simulink model "VSC_GFo_Fixed_Frequency_LCL"  (R2017a)
settings: Solver=ode1  StartTime=0.0  StopTime=15  FixedStep=Time_Step  MaxStep=1e-5  RelTol=1e-3
PreLoadFcn:
  | VSC_GFo_Init;
InitFcn:
  | VSC_GFo_Init;
undefined symbols (not defined in the file): fb, GRD00_H, GRD00_R, GRD00_TD, GRD00_TN, GRD00_Ub, L_1, L_2, R_1, R_2, Time_Step, VSC01_Delta_P_Time_Step, VSC01_Delta_P_Value
libraries: powerlib x14, Source_Lib x1, GFo_Lib x1
settings Model: Creator=Frederic_Colas  LastModifiedBy=Frederic_Colas
settings DataIOCC: SaveFormat=StructureWithTime
settings OptimizationCC: LifeSpan=inf
settings DebuggingCC: UnconnectedInputMsg=none  UnconnectedOutputMsg=none  UnconnectedLineMsg=none  SFExecutionAtInitializationDiag=none
settings HardwareCC: ProdBitPerSizeT=32  ProdBitPerPtrDiffT=32  ProdWordSize=32  ProdHWDeviceType=Specified
settings SimscapeCC: SimscapeNormalizeSystem=off

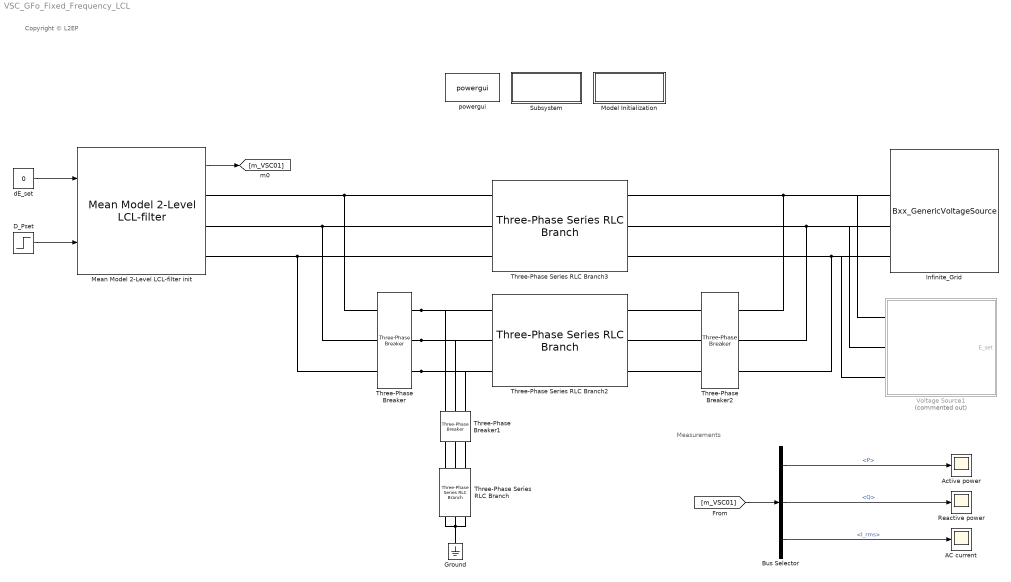
== system VSC_GFo_Fixed_Frequency_LCL ==
  note: Copyright © L2EP
  note: Measurements
  AC current : Scope
  Active power : Scope
  Bus Selector : BusSelector  OutputSignals=control.P,control.Q,control.VI.I_rms
  D_Pset : Step  Time=VSC01_Delta_P_Time_Step  After=VSC01_Delta_P_Value  SampleTime=0
  Ground : powerlib/Elements/Ground  LConnTagsString=a
  Infinite_Grid : Source_Lib/Bxx_GenericVoltageSource  SourceNature_str=INFINITE  fn=50  Sn=1e9  Un=400e3  LFpopup=Swing  P0=-778001534.1192  Q0=217439550.3985  V0_pu=1  U0=20000  Theta0_deg=0  H_s=5  DroopOnOff=on  R_percent=4  TN=1  TD=2
      settings: SourceProductName=VSC4SPS
  Mean Model 2-Level LCL-filter init : GFo_Lib/Mean Model 2-Level LCL-filter  fn=fn  Sn=VSC01_Sn  Pn=VSC01_Pn  Udcn=VSC01_Udc_n  Un1=VSC01_Un1  Un2=VSC01_Un2  Rt_pu=0.005  Lt_pu=0.15  Rm_pu=500  Lm_pu=500  Lf_pu=0.15  Rf_pu=0.005  Cf_pu=0.066  Tr_PLL=10e-3  Val_Freq_Support=on  Val_gamma=on  R_percent=4  Rv=0.009  W_TVR=60  I_thresh_pu=1  DX_DR=5  Kp_Rvi_pu=0.676  gainpopup=3  wc1=31.4159  mp1=0.0043  wc2=33.3  mp2=0.0033  wc3=2.5  mp3=0.04  T1=0.1210  T2=0.022  LFpopup=PQ  P0=0.79991  Q0=0.00012364  V0=0.99007  Theta0=15.6198  innercontrol=1  Kp_i=0.73/2  Ki_i=1.19/2  Kp_v=0.52  Ki_v=1.16  Kffv=1  Kffi=1  I_max=1.25
      settings: SourceProductName=VSC_Lib
  Model Initialization : Subsystem  mask(Model Functions){InitFcnX=VSC_GFo_Init;, prel=on, posl=off, inif=on, strf=off}
      mask prompts: InitFcnX "Initialisation"; prel "Preload Function"; posl "PostLoad Function"; inif "InitFcn"; strf "StartFcn"
      mask init:
      | currentBlock = gcb;
      | root = bdroot(currentBlock);
      | 
      | if ~strcmp(get_param(root,'BlockDiagramType'),'library')
      |     if prel==1
      |         set_param(root, 'PreLoadFcn', InitFcnX);
      |     else
      |         set_param(root, 'PreLoadFcn', '');
      |     end
      |     if inif==1
      |         set_param(root, 'InitFcn', InitFcnX);
      |     else
      |         set_param(root, 'InitFcn', '');
      |     end
      |     if strf==1
      |         set_param(root, 'StartFcn', InitFcnX);
      |     else
      |         set_param(root, 'StartFcn', '');
      |     end
      |     if posl==1
      |         set_param(root, 'PostLoadFcn', InitFcnX);
      |     else
      |         set_param(root, 'PostLoadFcn', '');
      |     end
      | end
      | 
      | pos = get_param(currentBlock, 'Position');
      | width = pos(3) - pos(1); height = pos(4) - pos(2);
      | txt = [ upper(root) '\n' '- InitFcn. . . . . '  get_param(root, 'InitFcn') ];
      settings: CopyFcn=set_param(gcb,'LinkStatus','none')
      mask Display:
      | %text(5, height*0.5, txt, 'horizontalAlignment', 'left', 'verticalAlignment', 'middle') ;
      | color('blue'),disp('Initialization Function\nParameters')
  Reactive power : Scope
  Subsystem : Subsystem
      settings: OpenFcn=LoadFlow_VSC
      mask Display: color('blue'),disp('Update Loadflow')
  Three-Phase Series RLC Branch : powerlib/Elements/Three-Phase Series RLC Branch  LConnTagsString=A|B|C  RConnTagsString=A|B|C  BranchType=R  Resistance=0.01  Inductance=1e-3  Capacitance=1e-6  Measurements=None
  Three-Phase Series RLC Branch2 : powerlib/Elements/Three-Phase Series RLC Branch  LConnTagsString=A|B|C  RConnTagsString=A|B|C  BranchType=RL  Resistance=R_2  Inductance=L_2  Capacitance=1e-6  Measurements=None
  Three-Phase Series RLC Branch3 : powerlib/Elements/Three-Phase Series RLC Branch  LConnTagsString=A|B|C  RConnTagsString=A|B|C  BranchType=RL  Resistance=R_1  Inductance=L_1  Capacitance=1e-6  Measurements=None
  Three-Phase Breaker : powerlib/Elements/Three-Phase Breaker  InitialState=closed  SwitchA=on  SwitchB=on  SwitchC=on  SwitchTimes=[1.5 4]  External=off  BreakerResistance=0.01  SnubberResistance=1e6  SnubberCapacitance=inf  Measurements=None
  Three-Phase Breaker1 : powerlib/Elements/Three-Phase Breaker  InitialState=open  SwitchA=on  SwitchB=on  SwitchC=on  SwitchTimes=[10 10.2]  External=off  BreakerResistance=0.01  SnubberResistance=1e6  SnubberCapacitance=inf  Measurements=None
  Three-Phase Breaker2 : powerlib/Elements/Three-Phase Breaker  InitialState=closed  SwitchA=on  SwitchB=on  SwitchC=on  SwitchTimes=[1.5 4]  External=off  BreakerResistance=0.01  SnubberResistance=1e6  SnubberCapacitance=inf  Measurements=None
  Voltage Source1 : Subsystem  Commented=on  mask(Fixed_source){fb=fb, Sc=1e9, Ub=GRD00_Ub, H_eq=GRD00_H, Droop=GRD00_R, TN=GRD00_TN, TD=GRD00_TD}
      mask prompts: fb "Nominal Frequency (Hz)"; Sc "Nominal Power (VA)"; Ub "Nominal Voltage (V)"; H_eq "Inertial Constant H (s)"; Droop "Droop Gain"; TN "Lead Time Constant"; TD "Lag Time Constant"
      mask init:
      | % Base values
      |     wb=2*pi*fb;
      |     Ib=Sc/(sqrt(3)*Ub);
      |     Vb=Ub/sqrt(3);
      |     e0=Vb;
      |     Theta_e0=0;
      |   
      | % Parameters
      |     R=Droop;
      mask DialogControl Container5 Prompt: Nominal Values
      mask DialogControl Container16 Prompt: Network Time Constants
  dE_set : Constant  Value=0
  powergui : powerlib/powergui  Priority=1  SimulationMode=Discrete  SampleTime=Time_Step  frequency=60  Iterations=50  frequencyindice=50  Pbase=1000000000  ErrMax=1e-4  UnitsV=kV  UnitsW=MW  buscounter=0  FunctionMessages=off  echomessages=off  EnableUseOfTLC=off  CurrentSourceSwitches=off  DisableSnubberDevices=off  DisableRonSwitches=off  DisableVfSwitches=off  DisplayEquations=off  SolverType=Tustin/Backward Euler (TBE)  Interpol=off  ExternalGateDelay=off  methode=off  Ts=100  x0status=blocks  SPID=on  SwTol=0  HookPort=off  RestoreLinks=warning  ResistiveCurrentMeasurement=off  Frange=[0:2:500]  Ylog=off  Xlog=on  ShowGrid=off  save=off  variable=ZData  structure=0  ZoomFFT=off  StartTime=0.0  cycles=1  DisplayStyle=1  fundamental=60  FreqAxis=off  MaxFrequency=1000  frequencyindicesteady=1  RmsSteady=1  display=off
  wires:
  dE_set/1 -> Mean Model 2-Level LCL-filter init/1
  Mean Model 2-Level LCL-filter init/1 -> [m_VSC01]
  Bus Selector/1 -> Active power/1  "<P>"
  Bus Selector/2 -> Reactive power/1  "<Q>"
  [m_VSC01] -> Bus Selector/1
  Bus Selector/3 -> AC current/1  "<I_rms>"
  D_Pset/1 -> Mean Model 2-Level LCL-filter init/2
  connections:
  Three-Phase Breaker/LConn1 -- Mean Model 2-Level LCL-filter init/RConn1 -- Three-Phase Series RLC Branch3/LConn1
  Three-Phase Breaker/LConn2 -- Mean Model 2-Level LCL-filter init/RConn2 -- Three-Phase Series RLC Branch3/LConn2
  Three-Phase Breaker/LConn3 -- Mean Model 2-Level LCL-filter init/RConn3 -- Three-Phase Series RLC Branch3/LConn3
  Three-Phase Breaker2/RConn2 -- Voltage Source1/RConn2 -- Infinite_Grid/RConn2 -- Three-Phase Series RLC Branch3/RConn2
  Three-Phase Series RLC Branch/RConn2 -- Three-Phase Series RLC Branch/RConn3 -- Ground/LConn1 -- Three-Phase Series RLC Branch/RConn1
  Three-Phase Breaker/RConn3 -- Three-Phase Series RLC Branch2/LConn3 -- Three-Phase Breaker1/RConn3
  Three-Phase Breaker2/RConn1 -- Voltage Source1/RConn1 -- Infinite_Grid/RConn1 -- Three-Phase Series RLC Branch3/RConn1
  Three-Phase Breaker2/RConn3 -- Voltage Source1/RConn3 -- Infinite_Grid/RConn3 -- Three-Phase Series RLC Branch3/RConn3
  Three-Phase Breaker/RConn1 -- Three-Phase Series RLC Branch2/LConn1 -- Three-Phase Breaker1/RConn1
  Three-Phase Breaker/RConn2 -- Three-Phase Series RLC Branch2/LConn2 -- Three-Phase Breaker1/RConn2
  Three-Phase Series RLC Branch/LConn3 -- Three-Phase Breaker1/LConn3
  Three-Phase Breaker1/LConn2 -- Three-Phase Series RLC Branch/LConn2
  Three-Phase Series RLC Branch2/RConn3 -- Three-Phase Breaker2/LConn3
  Three-Phase Series RLC Branch2/RConn2 -- Three-Phase Breaker2/LConn2
  Three-Phase Series RLC Branch/LConn1 -- Three-Phase Breaker1/LConn1
  Three-Phase Series RLC Branch2/RConn1 -- Three-Phase Breaker2/LConn1

== system VSC_GFo_Fixed_Frequency_LCL/Model Initialization ==

== system VSC_GFo_Fixed_Frequency_LCL/Subsystem ==

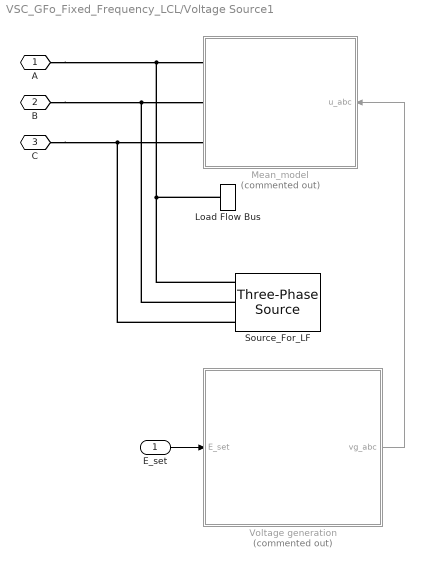
== system VSC_GFo_Fixed_Frequency_LCL/Voltage Source1 ==
  E_set : Inport
  Load Flow Bus : powerlib/Measurements/Load Flow Bus  LConnTagsString=a  Phases=single  Connectors=on one side  ID=BUS_1  Vbase=Ub  Vref=1  Vangle=0  VLF=1  VLFb=1  VLFc=1  angleLF=0  angleLFb=0  angleLFc=0
      settings: SourceProductName=Simscape Power Systems
  Mean_model : Subsystem  Commented=on
  Source_For_LF : powerlib/Electrical Sources/Three-Phase Source  InternalConnection=Yg  VoltagePhases=off  Voltage=(400000)*1  PhaseAngle=0  Voltage_phases=[25e3 25e3 25e3]/sqrt(3)  PhaseAngles_phases=[0 -120 +120]  Frequency=fb  NonIdealSource=on  SpecifyImpedance=off  Resistance=0  Inductance=0  ShortCircuitLevel=100e6  BaseVoltage=GRD00_Un  XRratio=7  BusType=swing  Pref=P0  Qref=Q0  Prefabc=[10e3, 10e3, 10e3]  Qrefabc=[0, 0, 0]  Qmin=-inf  Qmax=inf
  Voltage generation : Subsystem  Commented=on
  A : PMIOPort  Port=1  Side=Right
  B : PMIOPort  Port=2  Side=Right
  C : PMIOPort  Port=3  Side=Right
  wires:
  Voltage generation/1(vg_abc) -> Mean_model/1(u_abc)
  E_set/1 -> Voltage generation/1(E_set)
  connections:
  Load Flow Bus/LConn1 -- Source_For_LF/RConn1 -- A/RConn1 -- Mean_model/RConn1
  Source_For_LF/RConn2 -- B/RConn1 -- Mean_model/RConn2
  Source_For_LF/RConn3 -- C/RConn1 -- Mean_model/RConn3

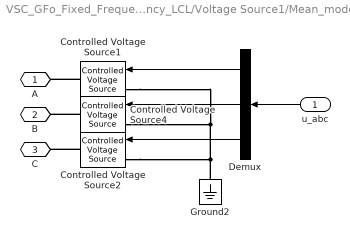
== system VSC_GFo_Fixed_Frequency_LCL/Voltage Source1/Mean_model ==
  u_abc : Inport
  Controlled Voltage Source1 : powerlib/Electrical Sources/Controlled Voltage Source  Initialize=on  Source_Type=AC  Amplitude=e0*sqrt(2)  Phase=0  Frequency=fb  Measurements=None
  Controlled Voltage Source2 : powerlib/Electrical Sources/Controlled Voltage Source  Initialize=on  Source_Type=AC  Amplitude=e0*sqrt(2)  Phase=-240  Frequency=fb  Measurements=None
  Controlled Voltage Source4 : powerlib/Electrical Sources/Controlled Voltage Source  Initialize=on  Source_Type=AC  Amplitude=e0*sqrt(2)  Phase=-120  Frequency=fb  Measurements=None
  Demux : Demux  Outputs=3
  Ground2 : powerlib/Elements/Ground  LConnTagsString=a
  A : PMIOPort  Port=1  Side=Right
  B : PMIOPort  Port=2  Side=Right
  C : PMIOPort  Port=3  Side=Right
  wires:
  Demux/1 -> Controlled Voltage Source1/1
  Demux/3 -> Controlled Voltage Source2/1
  Demux/2 -> Controlled Voltage Source4/1
  u_abc/1 -> Demux/1
  connections:
  Controlled Voltage Source1/RConn1 -- A/RConn1
  Controlled Voltage Source4/RConn1 -- B/RConn1
  Controlled Voltage Source2/RConn1 -- C/RConn1
  Ground2/LConn1 -- Controlled Voltage Source2/LConn1 -- Controlled Voltage Source1/LConn1 -- Controlled Voltage Source4/LConn1

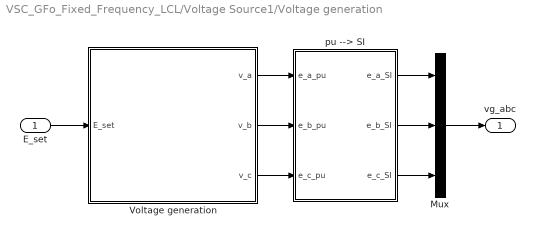
== system VSC_GFo_Fixed_Frequency_LCL/Voltage Source1/Voltage generation ==
  E_set : Inport
  Mux : Mux  Inputs=3
  Voltage generation : Subsystem
  pu --> SI : Subsystem
  vg_abc : Outport
  wires:
  E_set/1 -> Voltage generation/1(E_set)
  Voltage generation/2(v_b) -> pu --> SI/2(e_b_pu)
  Voltage generation/1(v_a) -> pu --> SI/1(e_a_pu)
  pu --> SI/2(e_b_SI) -> Mux/2
  pu --> SI/3(e_c_SI) -> Mux/3
  Mux/1 -> vg_abc/1
  Voltage generation/3(v_c) -> pu --> SI/3(e_c_pu)
  pu --> SI/1(e_a_SI) -> Mux/1

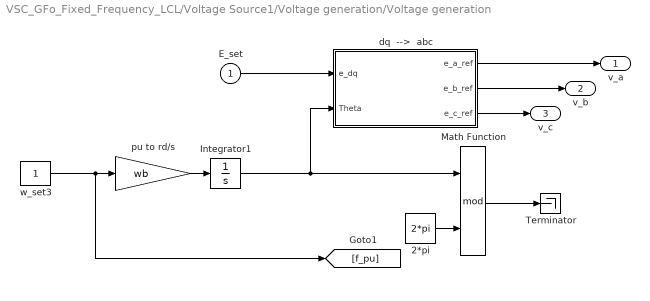
== system VSC_GFo_Fixed_Frequency_LCL/Voltage Source1/Voltage generation/Voltage generation ==
  E_set : Inport
  " pu to rd/s" : Gain  Gain=wb
  2*pi : Constant  Value=2*pi
  Integrator1 : Integrator
  Math Function : Math  Operator=mod  SaturateOnIntegerOverflow=on
  Terminator : Terminator
  "dq  -->  abc " : Subsystem
  w_set3 : Constant
  v_a : Outport
  v_b : Outport  Port=2
  v_c : Outport  Port=3
  wires:
  w_set3/1 -> " pu to rd/s"/1, [f_pu]
  E_set/1 -> "dq  -->  abc "/1(e_dq)
  "dq  -->  abc "/3(e_c_ref) -> v_c/1
  "dq  -->  abc "/2(e_b_ref) -> v_b/1
  "dq  -->  abc "/1(e_a_ref) -> v_a/1
  2*pi/1 -> Math Function/2
  Math Function/1 -> Terminator/1
  " pu to rd/s"/1 -> Integrator1/1
  Integrator1/1 -> Math Function/1, "dq  -->  abc "/2(Theta)

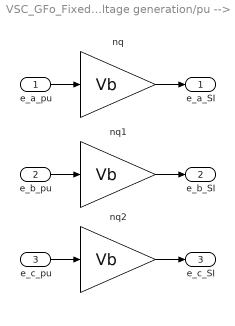
== system VSC_GFo_Fixed_Frequency_LCL/Voltage Source1/Voltage generation/pu --> SI ==
  e_a_pu : Inport
  e_b_pu : Inport  Port=2
  e_c_pu : Inport  Port=3
  nq : Gain  Gain=Vb
  nq1 : Gain  Gain=Vb
  nq2 : Gain  Gain=Vb
  e_a_SI : Outport
  e_b_SI : Outport  Port=2
  e_c_SI : Outport  Port=3
  wires:
  e_a_pu/1 -> nq/1
  nq1/1 -> e_b_SI/1
  e_c_pu/1 -> nq2/1
  nq/1 -> e_a_SI/1
  nq2/1 -> e_c_SI/1
  e_b_pu/1 -> nq1/1

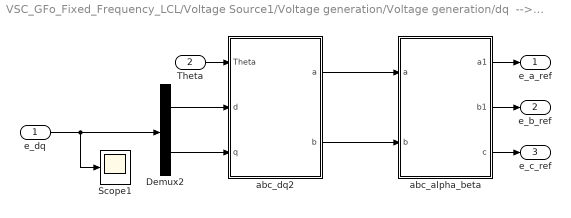
== system VSC_GFo_Fixed_Frequency_LCL/Voltage Source1/Voltage generation/Voltage generation/dq  -->  abc  ==
  e_dq : Inport
  Theta : Inport  Port=2
  Demux2 : Demux  Outputs=2
  Scope1 : Scope
  abc_alpha_beta : Subsystem
  abc_dq2 : Subsystem
  e_a_ref : Outport
  e_b_ref : Outport  Port=2
  e_c_ref : Outport  Port=3
  wires:
  abc_alpha_beta/1(a1) -> e_a_ref/1
  abc_alpha_beta/3(c) -> e_c_ref/1
  e_dq/1 -> Scope1/1, Demux2/1
  abc_alpha_beta/2(b1) -> e_b_ref/1
  Theta/1 -> abc_dq2/1(Theta)
  Demux2/2 -> abc_dq2/3(q)
  Demux2/1 -> abc_dq2/2(d)
  abc_dq2/2(b) -> abc_alpha_beta/2(b)
  abc_dq2/1(a) -> abc_alpha_beta/1(a)

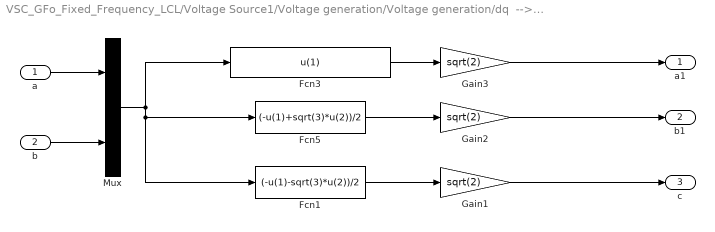
== system VSC_GFo_Fixed_Frequency_LCL/Voltage Source1/Voltage generation/Voltage generation/dq  -->  abc /abc_alpha_beta ==
  a : Inport
  b : Inport  Port=2
  Fcn1 : Fcn  Expr=(-u(1)-sqrt(3)*u(2))/2
  Fcn3 : Fcn  Expr=u(1)
  Fcn5 : Fcn  Expr=(-u(1)+sqrt(3)*u(2))/2
  Gain1 : Gain  Gain=sqrt(2)
  Gain2 : Gain  Gain=sqrt(2)
  Gain3 : Gain  Gain=sqrt(2)
  Mux : Mux  Inputs=2
  a1 : Outport
  b1 : Outport  Port=2
  c : Outport  Port=3
  wires:
  Gain3/1 -> a1/1
  Gain2/1 -> b1/1
  Gain1/1 -> c/1
  Fcn1/1 -> Gain1/1
  Fcn5/1 -> Gain2/1
  Fcn3/1 -> Gain3/1
  b/1 -> Mux/2
  a/1 -> Mux/1
  Mux/1 -> Fcn3/1, Fcn1/1, Fcn5/1

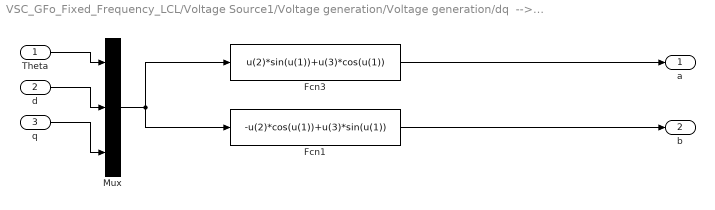
== system VSC_GFo_Fixed_Frequency_LCL/Voltage Source1/Voltage generation/Voltage generation/dq  -->  abc /abc_dq2 ==
  Theta : Inport
  d : Inport  Port=2
  q : Inport  Port=3
  Fcn1 : Fcn  Expr=-u(2)*cos(u(1))+u(3)*sin(u(1))
  Fcn3 : Fcn  Expr=u(2)*sin(u(1))+u(3)*cos(u(1))
  Mux : Mux  Inputs=3
  a : Outport
  b : Outport  Port=2
  wires:
  Mux/1 -> Fcn1/1, Fcn3/1
  Theta/1 -> Mux/1
  d/1 -> Mux/2
  q/1 -> Mux/3
  Fcn3/1 -> a/1
  Fcn1/1 -> b/1
